simulink model "teaching"  (R2016b)
settings: Solver=VariableStepAuto  StartTime=0.0  StopTime=25.0  MaxStep=1e-2  RelTol=1e-3
libraries: simulink x4
settings Model: Creator=nicol  LastModifiedBy=nicol

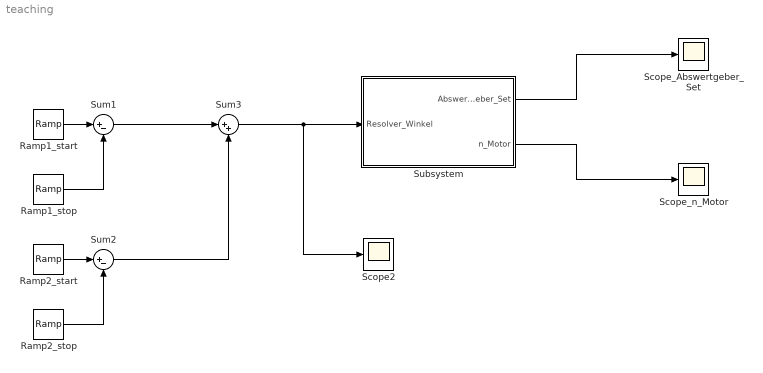
== system teaching ==
  Ramp1_start : simulink/Sources/Ramp  slope=1  start=6  X0=0
  Ramp1_stop : simulink/Sources/Ramp  slope=1  start=9  X0=0
  Ramp2_start : simulink/Sources/Ramp  slope=-1  start=13  X0=0
  Ramp2_stop : simulink/Sources/Ramp  slope=-1  start=19  X0=0
  Scope2 : Scope
  Scope_Abswertgeber_Set : Scope
  Scope_n_Motor : Scope
  Subsystem : Subsystem
  Sum1 : Sum  Inputs=|+-
  Sum2 : Sum  Inputs=|+-
  Sum3 : Sum  Inputs=|++
  wires:
  Ramp1_start/1 -> Sum1/1
  Ramp1_stop/1 -> Sum1/2
  Subsystem/1(Abswertgeber_Set) -> Scope_Abswertgeber_Set/1
  Subsystem/2(n_Motor) -> Scope_n_Motor/1
  Ramp2_start/1 -> Sum2/1
  Ramp2_stop/1 -> Sum2/2
  Sum1/1 -> Sum3/1
  Sum2/1 -> Sum3/2
  Sum3/1 -> Scope2/1, Subsystem/1(Resolver_Winkel)

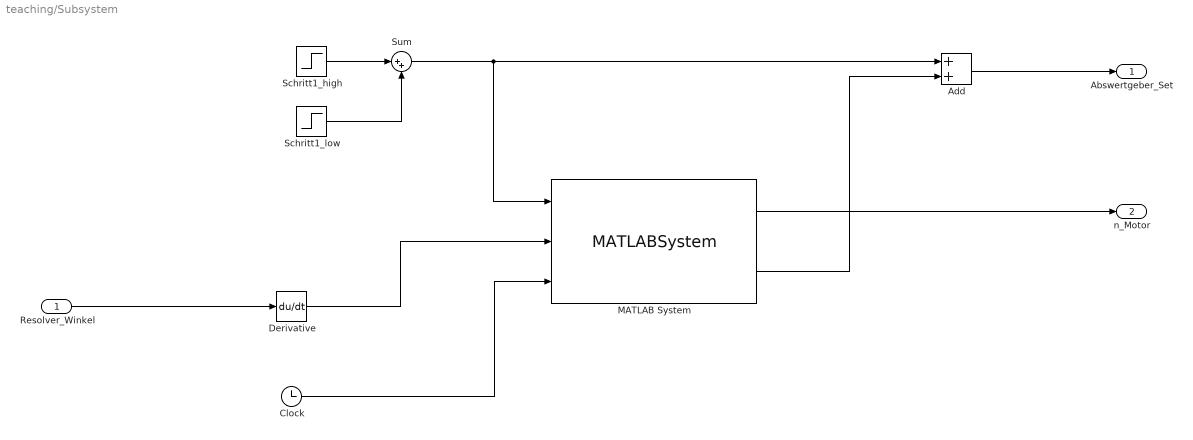
== system teaching/Subsystem ==
  Resolver_Winkel : Inport
  Add : Sum
  Clock : Clock
  Derivative : Derivative
  MATLAB System : MATLABSystem  System=Motorsteuerung2  SimulateUsing=Code generation
      mask Type: Motorsteuerung2
      mask Display:
      | disp('Motorsteuerung2');
      | port_label('input',1,'Schritt1');
      | port_label('input',2,'Resolver_Int');
      | port_label('input',3,'Clock');
      | port_label('output',1,'n_Motor');
      | port_label('output',2,'Abswertgeber_Set');
  Schritt1_high : Step  Time=0  SampleTime=0
  Schritt1_low : Step  Time=6  After=-1  SampleTime=0
  Sum : Sum  Inputs=|++
  Abswertgeber_Set : Outport
  n_Motor : Outport  Port=2
  wires:
  Schritt1_high/1 -> Sum/1
  Schritt1_low/1 -> Sum/2
  Sum/1 -> Add/1, MATLAB System/1
  Add/1 -> Abswertgeber_Set/1
  MATLAB System/1 -> n_Motor/1
  Clock/1 -> MATLAB System/3
  MATLAB System/2 -> Add/2
  Derivative/1 -> MATLAB System/2
  Resolver_Winkel/1 -> Derivative/1
